simulink model "PI_Electrico"  (R2022b)
settings: Solver=VariableStepAuto  StartTime=0.0  StopTime=5  RelTol=1e-3
libraries: fl_lib x8, nesl_utility x3, cstblocks x1
settings Model: Creator=Lambdax  LastModifiedBy=Lambdax

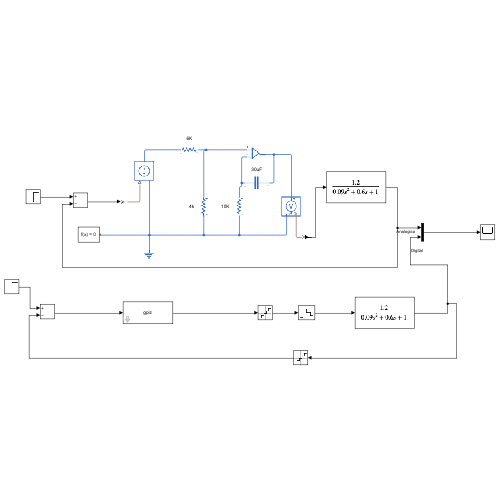
[thumbnail: Simulink's stored preview of the top-level diagram]
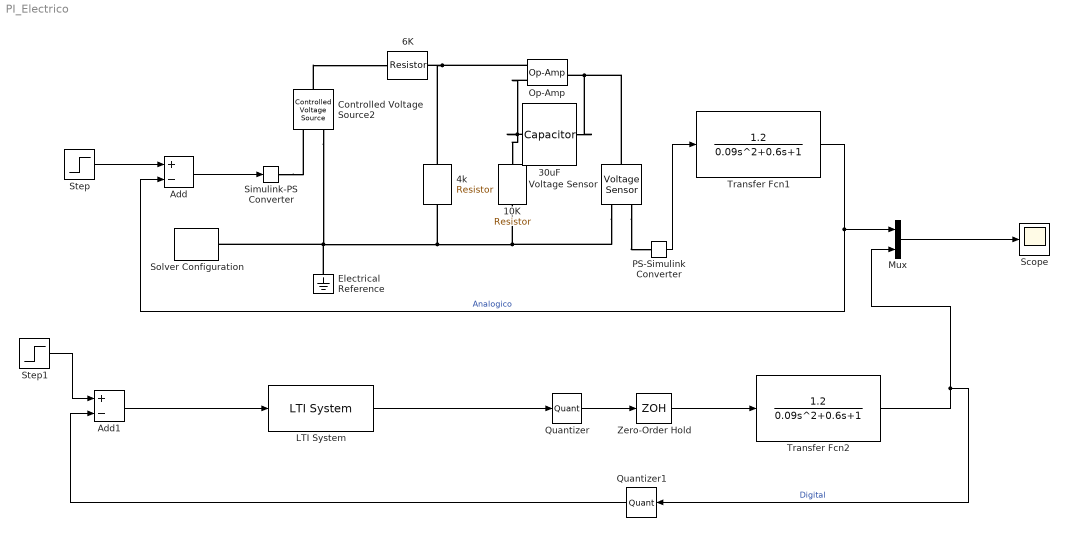
== system PI_Electrico ==
  10K : fl_lib/Electrical/Electrical Elements/Resistor  R=10000 Ohm  i_specify=off  i_priority=None  i=0 A  i_nominal_specify=off  i_nominal_unit=A  i_nominal_value=1  v_specify=off  v_priority=None  v=0 V  v_nominal_specify=off  v_nominal_unit=V  v_nominal_value=1
  30uF : fl_lib/Electrical/Electrical Elements/Capacitor  c=30e-6 F  r=1e-6 Ohm  g=0 1/Ohm  i_specify=off  i_priority=None  i=0 A  i_nominal_specify=off  i_nominal_unit=A  i_nominal_value=1  v_specify=off  v_priority=None  v=0 V  v_nominal_specify=off  v_nominal_unit=V  v_nominal_value=1  vc_specify=off  vc_priority=High  vc=0 V  vc_nominal_specify=off  vc_nominal_unit=V  vc_nominal_value=1
  4k : fl_lib/Electrical/Electrical Elements/Resistor  R=4000 Ohm  i_specify=off  i_priority=None  i=0 A  i_nominal_specify=off  i_nominal_unit=A  i_nominal_value=1  v_specify=off  v_priority=None  v=0 V  v_nominal_specify=off  v_nominal_unit=V  v_nominal_value=1
  6K : fl_lib/Electrical/Electrical Elements/Resistor  R=6000 Ohm  i_specify=off  i_priority=None  i=0 A  i_nominal_specify=off  i_nominal_unit=A  i_nominal_value=1  v_specify=off  v_priority=None  v=0 V  v_nominal_specify=off  v_nominal_unit=V  v_nominal_value=1
  Add : Sum  Inputs=+-
  Add1 : Sum  Inputs=+-
  Controlled Voltage Source2 : fl_lib/Electrical/Electrical Sources/Controlled Voltage Source
  Electrical Reference : fl_lib/Electrical/Electrical Elements/Electrical Reference
  LTI System : cstblocks/LTI System  sys=gpiz  IC=[]
  Mux : Mux  Inputs=2
  Op-Amp : fl_lib/Electrical/Electrical Elements/Op-Amp  outI_specify=off  outI_priority=None  outI=0 A  outI_nominal_specify=off  outI_nominal_unit=A  outI_nominal_value=1
  PS-Simulink Converter : nesl_utility/PS-Simulink Converter  PhysicalDomain=network_engine_domain  SubClassName=ps_output  LeftPortType=input  RightPortType=output  PseudoPeriodic=off  Frequencies=[]  VectorFormat=inherit  Unit=inherit  AffineConversion=off
  Quantizer : Quantizer  QuantizationInterval=0.001
  Quantizer1 : Quantizer  QuantizationInterval=0.001
  Scope : Scope
  Simulink-PS Converter : nesl_utility/Simulink-PS Converter  PhysicalDomain=network_engine_domain  SubClassName=ps_input  LeftPortType=input  RightPortType=output  PseudoPeriodic=off  Frequencies=[]  NoiseDistribution=none  NoiseParameters=[]  Unit=1  AffineConversion=off  FilteringAndDerivatives=provide  SimscapeFilterOrder=1  InputFilterTimeConstant=0.001  UdotUserProvided=0
  Solver Configuration : nesl_utility/Solver Configuration  PhysicalDomain=network_engine_domain  SubClassName=solver  LeftPortType=input  RightPortType=generic  Tones=[]  Harmonics=[]  SimulateNoise=off  Profile=off  UseLocalSampling=off  EnableSwitchedLinearOptims=on  FrequencyDomain=off  UseCCode=off  RelTol=0.001  AbsTol=0.001  MinStep=1e-09  ToWorkspace=off  RevertToSquareIcSolve=off  NumHomotopyIterations=100  PhasorMode=off  PhasorModeNumHarmonics=1  ConsistencySolver=NEWTON_XTOL_AFTER_FTOL  IndexReductionMethod=DerivativeReplacement  DoDC=off  ResidualTolerance=1e-09  ConsistencyTolSource=GLOBAL  ConsistencyAbsTol=0.001  ConsistencyRelTol=0.001  ConsistencyTolFactor=0.001  UseLocalSolver=off  LocalSolverChoice=NE_BACKWARD_EULER_ADVANCER  ResolveIndetEquations=on  FunctionEvalNumThread=1  LocalSolverSampleTime=0.001  DoFixedCost=off  MaxNonlinIter=3  MaxModeIter=2  ComputeImpulses=off  ImpulseIterations=2  LinearAlgebra=auto  LinearAlgebraNumThread=0  EquationFormulation=NE_TIME_EF  DelaysMemoryBudget=1024  AutomaticFiltering=on  FilteringTimeConstant=0.001  PartitionStorageMethod=AS_NEEDED  PartitionMemoryBudget=1024  PartitionMethod=ROBUST
  Step : Step  SampleTime=0
  Step1 : Step  SampleTime=0
  Transfer Fcn1 : TransferFcn  Numerator=[1.2]  Denominator=[0.09 0.6 1]
  Transfer Fcn2 : TransferFcn  Numerator=[1.2]  Denominator=[0.09 0.6 1]
  Voltage Sensor : fl_lib/Electrical/Electrical Sensors/Voltage Sensor
  Zero-Order Hold : ZeroOrderHold  SampleTime=0.22
  wires:
  Step/1 -> Add/1
  Add/1 -> Simulink-PS Converter/1
  PS-Simulink Converter/1 -> Transfer Fcn1/1
  Transfer Fcn1/1 -> Add/2, Mux/1  "Analogico"
  Mux/1 -> Scope/1
  LTI System/1 -> Quantizer/1
  Transfer Fcn2/1 -> Mux/2, Quantizer1/1  "Digital"
  Zero-Order Hold/1 -> Transfer Fcn2/1
  Quantizer/1 -> Zero-Order Hold/1
  Step1/1 -> Add1/1
  Add1/1 -> LTI System/1
  Quantizer1/1 -> Add1/2
  connections:
  Simulink-PS Converter/RConn1 -- Controlled Voltage Source2/RConn1
  Controlled Voltage Source2/LConn1 -- 6K/RConn1
  Op-Amp/LConn1 -- 4k/LConn1 -- 6K/LConn1
  Voltage Sensor/LConn1 -- 30uF/LConn1 -- Op-Amp/RConn1
  30uF/RConn1 -- 10K/LConn1 -- Op-Amp/LConn2
  Controlled Voltage Source2/RConn2 -- 4k/RConn1 -- Voltage Sensor/RConn2 -- 10K/RConn1 -- Electrical Reference/LConn1 -- Solver Configuration/RConn1
  Voltage Sensor/RConn1 -- PS-Simulink Converter/LConn1
